simulink model "PID_MEGA_SystemBlock"  (R2020a)
settings: Solver=FixedStepAuto  StartTime=0.0  StopTime=120  RelTol=1e-3  EnableMultiTasking=on
libraries: arduinolib x2, simulink x1, CommonBlocks x1
settings Model: SimulationMode=external  SILPILModeSetting=veronly  ExtModeTrigDuration=2  Creator=Jakub  LastModifiedBy=jakub
settings OptimizationCC: EnhancedBackFolding=on  PassReuseOutputArgsAs=Individual arguments  MaxStackSize=64  OptimizeBlockOrder=speed  DifferentSizesBufferReuse=on  OptimizationCustomize=off  EfficientTunableParamExpr=on
settings DebuggingCC: ParameterTunabilityLossMsg=error
settings HardwareCC: ProdBitPerInt=16  ProdBitPerPointer=16  ProdBitPerSizeT=16  ProdBitPerPtrDiffT=16  ProdLargestAtomicFloat=None  ProdWordSize=8  ProdHWDeviceType=Atmel->AVR
settings SFSimCC: MATLABDynamicMemAlloc=off  CustomCodeUndefinedFunction=UseInterfaceOnly
settings RTWCC: SystemTargetFile=ert.tlc  HardwareBoard=Arduino Mega 2560  TLCOptions=-aInlineSetEventsForThisBaseRateFcn=TLC_FALSE -aSuppressMultiTaskScheduler=TLC_FALSE -aRateBasedStepFcn=1  TemplateMakefile=ert_default_tmf  GenerateReport=on  Toolchain=Arduino AVR  BuildConfiguration=Faster Runs  IncludeHyperlinkInReport=on  LaunchReport=on  GenerateTraceInfo=on  GenerateTraceReport=on  GenerateTraceReportSl=on  GenerateTraceReportSf=on  GenerateTraceReportEml=on
settings CodeAppCC: ForceParamTrailComments=on  IgnoreCustomStorageClasses=off  OperatorAnnotations=on  SimulinkDataObjDesc=on  SFDataObjDesc=on  InsertBlockDesc=on
settings ERTTargetCC: SupportContinuousTime=on  SupportVariableSizeSignals=on  ExtModeStaticAllocSize=2048

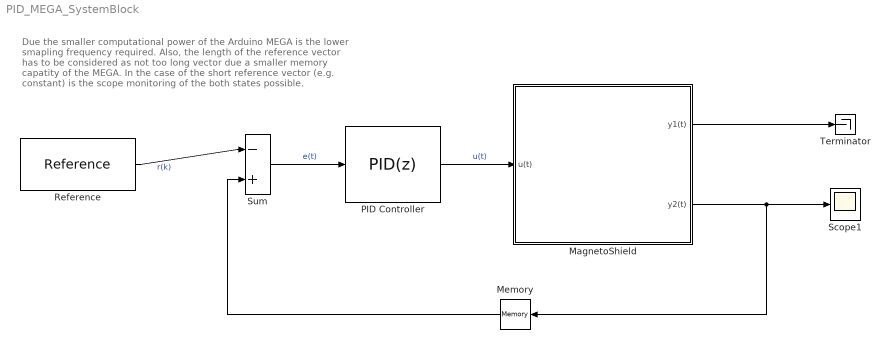
== system PID_MEGA_SystemBlock ==
  note: Due the smaller computational power of the Arduino MEGA is the
      | lower smapling frequency required.
      | Also, the length of the reference vector has to be considered
      | as not too long vector due a smaller memory capatity of the MEGA.
      |
      | In the case of the short reference vector (e.g. constant) is the scope
      | monitoring of the both states possible.
  MagnetoShield : Subsystem  AncestorBlock=MagnetoLibrary/MagnetoShield  mask{Board=UNO/MEGA, PositionType=Distance [mm], chackbox=on, Ts=-1}
      mask prompts: Board "Type of the Arduino board"; PositionType "Position measured in:"; chackbox "Execute calibration at the biginning of the simulation"; Ts "Sampling period [s]"
      mask help:
      | The block represents MagnetoShield system. On the input is a control signal in the form of voltage expected (values in the range 0 - 12 V).
      | Outputs are system states - Position (y1) and Current (y2). The position is possible to measure in milimeters or in percent.
      | In the case of the closed loop control, on the feedback signals to use 'Memory' block is recomended.
      mask init:
      | mask_popup = get_param(gcb,'Board'); % which popup is choosen
      | % path to the I2C Write block
      | system = gcb;
      | way = strcat(system,'/ActuatorWrite');
      | % set Module based on Arduino type
      | if strcmp(mask_popup(1),'U')
      |     set_param(way,'Board','UNO/MEGA'); % Uno/Mega - module 0
      | elseif strcmp(mask_popup(1),'D')
      |     set_param(way,'Board','DUE'); % Due - module 1
      | end
      settings: CopyFcn=set_param(gcb, 'LinkStatus', 'inactive')
      mask TypeOptions Board: UNO/MEGA | DUE
      mask TypeOptions PositionType: Distance [mm] | Percents [%]
      mask DialogControl DescGroupVar Prompt: MagnetoShield block
      mask DialogControl ParameterGroupVar Prompt: Arduino board
      mask DialogControl Container5 Prompt: Parameters
      mask Display: image('assets\MagnetoFig\MagnetoShield.svg');
  Memory : Memory  InheritSampleTime=on
  PID Controller : simulink/Continuous/PID Controller  Controller=PID  Form=Ideal  TimeDomain=Discrete-time  UseExternalTs=off  SampleTime=-1  IntegratorMethod=Forward Euler  FilterMethod=Forward Euler  ControllerParametersSource=internal  P=4  I=1/0.2  D=0.03  UseFilter=off  N=100  TunerSelectOption=Transfer Function Based (PID Tuner App)  InitialConditionSource=internal  InitialConditionForIntegrator=0  InitialConditionForFilter=0  DifferentiatorICPrevScaledInput=0  ExternalReset=none  TrackingMode=off  Kt=1  LimitOutput=on  UpperSaturationLimit=12  LowerSaturationLimit=0  LinearizeAsGain=on  AntiWindupMode=back-calculation  Kb=0.1  POutMin=[]  POutMax=[]  IOutMin=[]  IOutMax=[]  DOutMin=[]  DOutMax=[]  NOutMin=[]  NOutMax=[]  SumOutMin=[]  SumOutMax=[]  SaturationOutMin=[]  SaturationOutMax=[]  PParamMin=[]  PParamMax=[]  IParamMin=[]  IParamMax=[]  DParamMin=[]  DParamMax=[]  NParamMin=[]  NParamMax=[]  KbParamMin=[]  KbParamMax=[]  KtParamMin=[]  KtParamMax=[]  KbOutMin=[]  KbOutMax=[]  KtOutMin=[]  KtOutMax=[]  IntegratorOutMin=[]  IntegratorOutMax=[]  FilterOutMin=[]  FilterOutMax=[]  SumI1OutMin=[]  SumI1OutMax=[]  SumI2OutMin=[]  SumI2OutMax=[]  SumI3OutMin=[]  SumI3OutMax=[]  SumI4OutMin=[]  SumI4OutMax=[]  SumDOutMin=[]  SumDOutMax=[]  DifferentiatorOutMin=[]  DifferentiatorOutMax=[]  FilterDiffOutCoefMin=[]  FilterDiffOutCoefMax=[]  ReciprocalOutMin=[]  ReciprocalOutMax=[]  SumDenOutMin=[]  SumDenOutMax=[]  SumNumOutMin=[]  SumNumOutMax=[]  DivideOutMin=[]  DivideOutMax=[]  UdiffTsProdOutMin=[]  UdiffTsProdOutMax=[]  NTsProdOutMin=[]  NTsProdOutMax=[]  UintegralTsProdOutMin=[]  UintegralTsProdOutMax=[]  UngainTsProdOutMin=[]  UngainTsProdOutMax=[]  IntegratorContinuousStateAttributes=''  IntegratorStateMustResolveToSignalObject=off  IntegratorRTWStateStorageClass=Auto  FilterContinuousStateAttributes=''  FilterStateMustResolveToSignalObject=off  FilterRTWStateStorageClass=Auto  ParallelPVariant=Passthrough  IdealPVariant=InternalParameters  IVariant=InternalParameters  DVariant=InternalParameters  IntegratorVariant=Discrete  SatVariant=Enabled  AWVariant=BackCalculation  PCopyVariant=Disabled  TRVariant=Disabled  FdbkBlocksVariant=Forward  IdealPFdbkVariant=Disabled  SatFdbkVariant=Disabled  DerivativeFilterVariant=Differentiator  NVariant=Passthrough  NCopyVariant=Disabled_SignalSpec  FilterICVariant=InternalICsDifferentiator  IntegratorICVariant=InternalICs  ExternalResetVariant=Disabled  TRSumVariant=Passthrough  SumFdbkVariant=Disabled  SumVariant=Sum_PID  TsampFilterVariant=InternalTs  TsampNgainVariant=Passthrough  TsampIntegralVariant=Passthrough
  Reference : CommonBlocks/Reference  RefVect=[17 13 15 14 13 12 15]  AtTheEnd=Stop simulation  Reps=5  SectLen=2000  OffsetTime=0  Ts=0.002
      settings: SourceProductName=AutomationShield
  Scope1 : Scope
  Sum : Sum  Inputs=|-+
  Terminator : Terminator
  wires:
  Sum/1 -> PID Controller/1  "e(t)"
  PID Controller/1 -> MagnetoShield/1(u(t))  "u(t)"
  MagnetoShield/1(y1(t)) -> Terminator/1
  MagnetoShield/2(y2(t)) -> Scope1/1, Memory/1
  Memory/1 -> Sum/2
  Reference/1 -> Sum/1  "r(k)"

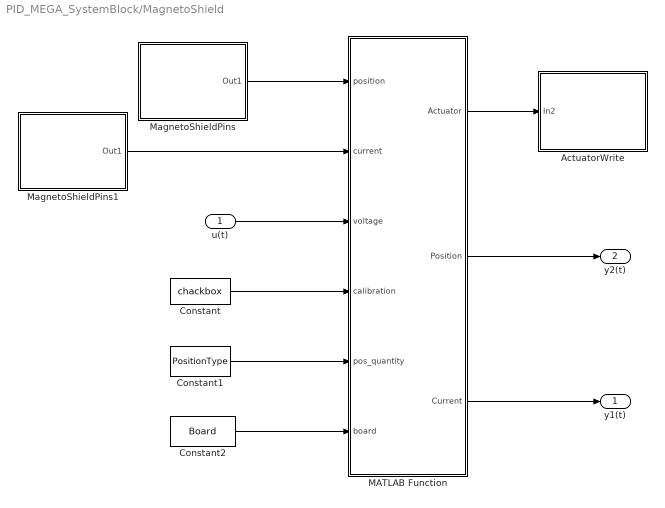
== system PID_MEGA_SystemBlock/MagnetoShield ==
  u(t) : Inport
  ActuatorWrite : Subsystem  AncestorBlock=MagnetoLibrary/ActuatorWrite  mask{Board=UNO/MEGA, Units=Volts}
      mask prompts: Board "Type of the Arduino board"; Units "Input unite"
      mask help:
      | ActuatorWrite block allows to set desired voltage value on the electromagnet. The desired value can be expresed as voltage, percentage of maximal possible voltage or as a value of the magnetic field in Gausses as well.
      | This block converts input control signal into suficient form (16-bit number) and writes the information on the MCP4725-DAC converter.
      | Maximal voltage range: 0-12 V
      mask init:
      | mask_popup = get_param(gcb,'Board'); % which popup is choosen
      | % path to the I2C Write block
      | system = gcb;
      | way = strcat(system,'/I2C Write UNO');
      | % set Module based on Arduino type
      | if strcmp(mask_popup(1),'U')
      |     set_param(way,'I2CModule','0'); % Uno/Mega - module 0
      | elseif strcmp(mask_popup(1),'D')
      |     set_param(way,'I2CModule','1'); % Due - module 1
      | end
      settings: CopyFcn=set_param(gcb, 'LinkStatus', 'inactive')
      mask TypeOptions Board: UNO/MEGA | DUE
      mask TypeOptions Units: Volts | Percents | DAC levels
      mask DialogControl DescGroupVar Prompt: ActuatorWrite block
      mask Display: image('assets\MagnetoFig\ActuatorWrite.svg');
  Constant : Constant  Value=chackbox  SampleTime=Ts
  Constant1 : Constant  Value=PositionType  SampleTime=Ts
  Constant2 : Constant  Value=Board  SampleTime=Ts
  MATLAB Function : MATLAB Function  TreatAsAtomicUnit=on
  MagnetoShieldPins : Subsystem  AncestorBlock=MagnetoLibrary/MagnetoShieldPins  mask{PIN=Hall sensor pin (A3), sampling=Ts}
      mask prompts: PIN "Choose pin"; sampling "Sampling period [s]"
      mask help:
      | User can choose a pin on which the data should be processed.
      | >Hall sensor pin - data about the possition of the levitating magnet.
      | >Voltage pin - voltage on the electromagnet
      | >Current pin - current crossing the electromagnet
      | >Reference pin - data from potentiometer, used as adjustable analog reference
      | (output = double)
      mask init:
      | letter = PIN;
      | if letter==1
      | path='assets\MagnetoFig\Pins\hpin.svg';
      | elseif letter==2
      | path='assets\MagnetoFig\Pins\vpin.svg';
      | elseif letter==3
      | path='assets\MagnetoFig\Pins\cpin.svg';
      | else
      | path='assets\MagnetoFig\Pins\ppin.svg';    
      | end
      settings: CopyFcn=set_param(gcb, 'LinkStatus', 'inactive')
      mask TypeOptions PIN: Hall sensor pin (A3) | Voltage pin (A1) | Current pin (A2) | Reference pin (A0)
      mask Callback PIN:
      | mask_popup = get_param(gcb,'PIN'); % which popup is choosen
      | % path to the I2C Write block
      | system = gcb;
      | way = strcat(system,'/Analog Input');
      | % set Module based on Arduino type
      | if strcmp(mask_popup(1),'H')
      |     set_param(way,'pinNumber','3'); % Uno/Mega - module 0
      | elseif strcmp(mask_popup(1),'V')
      |     set_param(way,'pinNumber','1'); % Due - module 1
      | elseif strcmp(mask_popup(1),'C')
      |     set_param(way,'pinNumber','2'); % Due - module 1
      | elseif strcmp(mask_popup(1),'R')
      |     set_param(way,'pinNumber','0'); % Due - module 11
      | end
      mask DialogControl DescGroupVar Prompt: MagnetoShieldPins block
      mask Display: image(path);
  MagnetoShieldPins1 : Subsystem  AncestorBlock=MagnetoLibrary/MagnetoShieldPins  mask{PIN=Current pin (A2), sampling=Ts}
      mask prompts: PIN "Choose pin"; sampling "Sampling period [s]"
      mask help:
      | User can choose a pin on which the data should be processed.
      | >Hall sensor pin - data about the possition of the levitating magnet.
      | >Voltage pin - voltage on the electromagnet
      | >Current pin - current crossing the electromagnet
      | >Reference pin - data from potentiometer, used as adjustable analog reference
      | (output = double)
      mask init: same as PID_MEGA_SystemBlock/MagnetoShield/MagnetoShieldPins
      settings: CopyFcn=set_param(gcb, 'LinkStatus', 'inactive')
      mask TypeOptions PIN: Hall sensor pin (A3) | Voltage pin (A1) | Current pin (A2) | Reference pin (A0)
      mask Callback PIN:
      | mask_popup = get_param(gcb,'PIN'); % which popup is choosen
      | % path to the I2C Write block
      | system = gcb;
      | way = strcat(system,'/Analog Input');
      | % set Module based on Arduino type
      | if strcmp(mask_popup(1),'H')
      |     set_param(way,'pinNumber','3'); % Uno/Mega - module 0
      | elseif strcmp(mask_popup(1),'V')
      |     set_param(way,'pinNumber','1'); % Due - module 1
      | elseif strcmp(mask_popup(1),'C')
      |     set_param(way,'pinNumber','2'); % Due - module 1
      | elseif strcmp(mask_popup(1),'R')
      |     set_param(way,'pinNumber','0'); % Due - module 11
      | end
      mask DialogControl DescGroupVar Prompt: MagnetoShieldPins block
      mask Display: image(path);
  y1(t) : Outport  VectorParamsAs1DForOutWhenUnconnected=off
  y2(t) : Outport  Port=2  VectorParamsAs1DForOutWhenUnconnected=off
  wires:
  MATLAB Function/3(Current) -> y1(t)/1
  Constant2/1 -> MATLAB Function/6(board)
  Constant1/1 -> MATLAB Function/5(pos_quantity)
  Constant/1 -> MATLAB Function/4(calibration)
  MagnetoShieldPins1/1(Out1) -> MATLAB Function/2(current)
  u(t)/1 -> MATLAB Function/3(voltage)
  MATLAB Function/2(Position) -> y2(t)/1
  MagnetoShieldPins/1(Out1) -> MATLAB Function/1(position)
  MATLAB Function/1(Actuator) -> ActuatorWrite/1(In2)

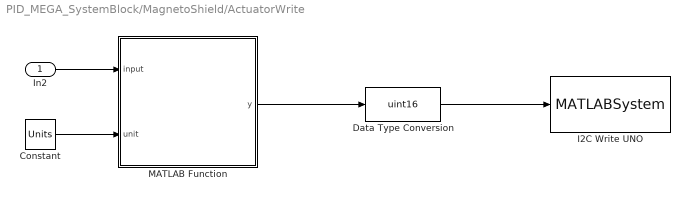
== system PID_MEGA_SystemBlock/MagnetoShield/ActuatorWrite ==
  In2 : Inport
  Constant : Constant  Value=Units
  Data Type Conversion : DataTypeConversion  OutDataTypeStr=uint16
  I2C Write UNO : MATLABSystem  AncestorBlock=arduinolib/I2C Write  InitFcn=|  System=codertarget.arduinobase.internal.arduinoI2CWrite  I2CModule=0  Mode=Master  SlaveAddress=96  SlaveByteOrder=BigEndian  Direction=Transmitter  RegisterAddressMode=off  RegisterAddress=0  SlaveDataType=uint8  DataLength=1  NoAck=off  RepeatedStart=off  OutputStatus=off  blockPlatform=ARDUINO
      | codertarget.arduinobase.blocks.registerI2CBlock(gcbh);
      | codertarget.arduinobase.blocks.arduinoBlockInitFcnCallback(gcbh);
      mask Type: I2C Write
      mask Display:
      | color('white');
      | plot([100,100,100,100],[100,100,100,100]);
      | plot([0,0,0,0],[0,0,0,0]);
      | color('blue');
      | text(99, 92, 'ARDUINO', 'horizontalAlignment', 'right');
      | color('black');
      | text(50,60,'\fontsize{12}\bfI2C','texmode','on','horizontalAlignment','center','verticalAlignment','middle');
      | text(50,40,'\fontsize{10}\bfMaster Write','texmode','on','horizontalAlignment','center','verticalAlignment','middle');
      | text(50,15,'Slave: 0x60' ,'horizontalAlignment', 'center');
      | port_label('input',1,'Data');
  MATLAB Function : MATLAB Function  TreatAsAtomicUnit=on
  wires:
  In2/1 -> MATLAB Function/1(input)
  Constant/1 -> MATLAB Function/2(unit)
  Data Type Conversion/1 -> I2C Write UNO/1
  MATLAB Function/1(y) -> Data Type Conversion/1

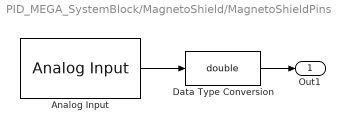
== system PID_MEGA_SystemBlock/MagnetoShield/MagnetoShieldPins ==
  Analog Input : arduinolib/Analog Input  pinNumber=3  ReadResultsOnly=off  ConversionTriggerSource=Software  ExternalTriggerType=uint32(0)  OutputDataType=uint16  EnableConversionCompleteNotify=off  EnableOuputStatus=off  SampleTime=sampling  blockPlatform=arduino
  Data Type Conversion : DataTypeConversion  OutDataTypeStr=double
  Out1 : Outport  VectorParamsAs1DForOutWhenUnconnected=off
  wires:
  Analog Input/1 -> Data Type Conversion/1
  Data Type Conversion/1 -> Out1/1

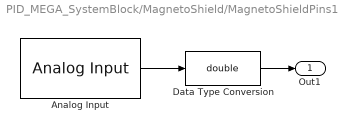
== system PID_MEGA_SystemBlock/MagnetoShield/MagnetoShieldPins1 ==
  Analog Input : arduinolib/Analog Input  pinNumber=2  ReadResultsOnly=off  ConversionTriggerSource=Software  ExternalTriggerType=uint32(0)  OutputDataType=uint16  EnableConversionCompleteNotify=off  EnableOuputStatus=off  SampleTime=sampling  blockPlatform=arduino
  Data Type Conversion : DataTypeConversion  OutDataTypeStr=double
  Out1 : Outport  VectorParamsAs1DForOutWhenUnconnected=off
  wires:
  Analog Input/1 -> Data Type Conversion/1
  Data Type Conversion/1 -> Out1/1

== matlab function PID_MEGA_SystemBlock/MagnetoShield/ActuatorWrite/MATLAB Function ==
  data: input input; y output; unit input
function y = fcn(input,unit)

if unit==1 % voltage
    y = 4095/12*input;
elseif unit==2 % percents
    y = 4095/100*input;
elseif unit==3 % dac levels
    y = input;
else
     y = 0; % needed instance
end
% secures that 12-bit number will not overcross a size boundary
if y>4095
    y=4095;
elseif y<0
    y=0;
end

end

== matlab function PID_MEGA_SystemBlock/MagnetoShield/MATLAB Function ==
  data: position input; Actuator output; current input; Position output; voltage input; calibration input; Current output; pos_quantity input; board input
function [Actuator,Position,Current] = fcn(position,current,voltage,calibration,pos_quantity,board)
persistent adcMAX adcMIN p_d1 p_d2 counter calib ARES3V3 A1302_SENSITIVITY;
if isempty(counter)
         p_d1 = 3.233100;
         p_d2 = 0.220571;
         counter = 0;
         adcMAX = 300;
         adcMIN = 300;
         calib = calibration;
         A1302_SENSITIVITY = 769.23;
         if board==1                 % choose board
            ARES3V3 = 3.3/1023;     % UNO
         else 
            ARES3V3 = 3.3/4095;     % DUE
         end
end
% CALIBRATION PHASE
if calib == 1
    % Minimal ADC level measured on the hall sensor
    if counter<=500
        Actuator = 0;
        if position<adcMIN
            adcMIN = position;
        end
    % Maximal ADC level measured on the hall sensor    
    elseif counter>500 && counter<=1000
        Actuator = 12;
        if position>adcMAX
            adcMAX = position; 
        end
    % Calibration calculations
    else
        Actuator = 0;
        p_d2 = log(17/12)/log((2.5-adcMIN*ARES3V3)*A1302_SENSITIVITY/((2.5-adcMAX*ARES3V3)*A1302_SENSITIVITY));
        p_d1 = 12/((2.5-adcMAX*ARES3V3)*A1302_SENSITIVITY)^p_d2;
        % Time 500 samples to settle down the magnet
        if counter>1500
            calib = 0;
        end
    end
    Position = 0;   % default outputs during calibration
    Current = 0;
    counter = counter+1;
% CONTROL PHASE
elseif calib == 0
    Actuator = voltage;
    % position measured in:
    if pos_quantity==2  % percents
        Position = (position-adcMIN)*100/(adcMAX-adcMIN);
    else            % distance
        gauss = (2.5-position*ARES3V3)*A1302_SENSITIVITY;
        Position = p_d1*gauss^p_d2;
    end
    % current measurement
    Current = current*ARES3V3*33.333333; %Igain = 33.333333
% ERROR SIGNALIZATION    
else
    Actuator = 42;
    Position = 42;
    Current = 42;
end
